simulink model "dianliuhuan"  (Simulink 8.5)
settings: Solver=ode23tb  StartTime=0.0  StopTime=5  RelTol=1e-3
libraries: powerlib x14, powerlib_extras x2
settings Model: Creator=Administrator  LastModifiedBy=佳君
settings DebuggingCC: SolverPrmCheckMsg=warning  FcnCallInpInsideContextMsg=UseLocalSettings  StrictBusMsg=Warning

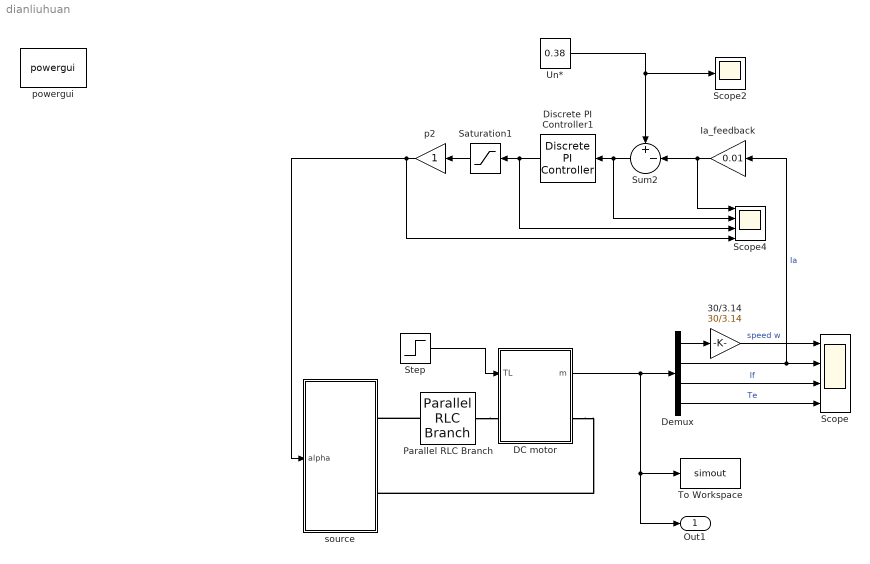
== system dianliuhuan ==
  30/3.14 : Gain  Gain=30/3.14
  DC motor : Subsystem
  Demux : Demux
  Discrete PI Controller1 : powerlib_extras/Discrete  Control Blocks/Discrete PI Controller  Kp=01  Ki=6  Par_Limits=[1e6 -1e6]  Init=0  Ts=50e-6
  Ia_feedback : Gain  Gain=0.01
  Parallel RLC Branch : powerlib/Elements/Parallel RLC Branch  LConnTagsString=a  RConnTagsString=__new0  BranchType=L  Resistance=1  Inductance=1e-3  SetiL0=off  InitialCurrent=0  Capacitance=1e-6  Setx0=off  InitialVoltage=0  Measurements=Branch voltage and current
  Saturation1 : Saturate  UpperLimit=10  LowerLimit=-10
  Scope : Scope  NumInputPorts=4
      settings: TimeRange=5  YMin=-0.1290027482477591~0~0.9166666666665609~0  YMax=2000~600~0.9166666666667626~1000
  Scope2 : Scope
      settings: YMin=0  YMax=13  SaveName=ScopeData2
  Scope4 : Scope  NumInputPorts=4
      settings: TimeRange=5  YMin=0~-5~-12~0  YMax=5.5~0.5~1~0.3  SaveName=ScopeData4
  Step : Step  Time=2  Before=50  After=100  SampleTime=0
  Sum2 : Sum  Inputs=+-|
  To Workspace : ToWorkspace  VariableName=simout  SaveFormat=Structure  SampleTime=-1
  Un* : Constant  Value=0.38
  p2 : Gain
  powergui : powerlib/powergui  Priority=1  SimulationMode=Continuous  SolverType=Tustin/Backward Euler (TBE)  SampleTime=50e-6  frequency=60  SPID=off  DisableSnubberDevices=off  DisableRonSwitches=off  DisableVfSwitches=off  SwTol=0  DisplayEquations=off  Interpol=off  methode=off  Ts=0  FunctionMessages=off  echomessages=off  HookPort=off  EnableUseOfTLC=off  x0status=blocks  frequencyindice=0  Pbase=100e6  ErrMax=1e-4  Iterations=50  UnitsV=kV  UnitsW=MW  buscounter=0  RestoreLinks=warning  ResistiveCurrentMeasurement=off  Frange=[0:2:500]  Ylog=off  Xlog=on  ShowGrid=off  save=off  variable=ZData  structure=0  ZoomFFT=on  StartTime=0.0  cycles=1  DisplayStyle=1  fundamental=60  FreqAxis=off  MaxFrequency=1000  frequencyindicesteady=1  RmsSteady=1  display=off
  source : Subsystem
  Out1 : Outport
  wires:
  DC motor/1(m) -> Demux/1, Out1/1, To Workspace/1
  Demux/2 -> Ia_feedback/1, Scope/2  "Ia"
  Demux/3 -> Scope/3  "If"
  Demux/4 -> Scope/4  "Te"
  Demux/1 -> 30/3.14/1
  30/3.14/1 -> Scope/1  "speed w"
  Step/1 -> DC motor/1(TL)
  Ia_feedback/1 -> Sum2/2, Scope4/1
  Sum2/1 -> Scope4/2, Discrete PI Controller1/1
  Saturation1/1 -> p2/1
  p2/1 -> Scope4/4, source/1(alpha)
  Un*/1 -> Sum2/1, Scope2/1
  Discrete PI Controller1/1 -> Scope4/3, Saturation1/1
  connections:
  Parallel RLC Branch/LConn1 -- source/RConn1
  Parallel RLC Branch/RConn1 -- DC motor/LConn1
  DC motor/RConn1 -- source/RConn2

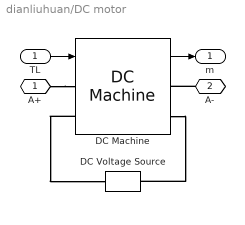
== system dianliuhuan/DC motor ==
  TL : Inport
  DC Machine : powerlib/Machines/DC Machine  PresetModel=No  MechanicalLoad=Torque TL  FieldType=Wound  ShowDetailedParameters=on  MeasurementBus=off  RLa=[0.6 0.012]  RLf=[240 120]  Laf=1.8  MachineConstant=Torque constant (N.m/A)  Ke=1.8  Kt=1.8  J=1  Bm=0  Tf=0  w0=0  Ifinit=0  TsPowergui=0  TsBlock=-1
  DC Voltage Source : powerlib/Electrical Sources/DC Voltage Source  Amplitude=220  Measurements=None
  A+ : PMIOPort  Port=1  Side=Left
  A- : PMIOPort  Port=2  Side=Right
  m : Outport
  wires:
  TL/1 -> DC Machine/1
  DC Machine/1 -> m/1
  connections:
  DC Machine/LConn2 -- DC Voltage Source/RConn1
  DC Machine/RConn2 -- DC Voltage Source/LConn1
  A+/RConn1 -- DC Machine/LConn1
  A-/RConn1 -- DC Machine/RConn1

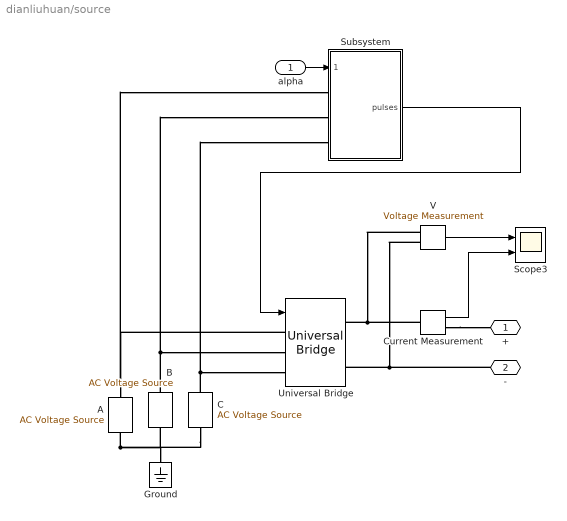
== system dianliuhuan/source ==
  alpha : Inport
  A : powerlib/Electrical Sources/AC Voltage Source  Amplitude=220  Phase=0  Frequency=50  SampleTime=0  Measurements=Voltage
  B : powerlib/Electrical Sources/AC Voltage Source  Amplitude=220  Phase=240  Frequency=50  SampleTime=0  Measurements=Voltage
  C : powerlib/Electrical Sources/AC Voltage Source  Amplitude=220  Phase=120  Frequency=50  SampleTime=0  Measurements=Voltage
  Current Measurement : powerlib/Measurements/Current Measurement  PhasorSimulation=off  OutputType=Complex  PSBequivalent=0
  Ground : powerlib/Elements/Ground  LConnTagsString=a
  Scope3 : Scope  NumInputPorts=2
      settings: YMin=-25~0  YMax=400~525
  Subsystem : Subsystem
  Universal Bridge : powerlib/Power Electronics/Universal Bridge  Arms=3  SnubberResistance=1e5  SnubberCapacitance=inf  Device=Thyristors  Ron=1e-3  Lon=0  ForwardVoltages="[  0  0  ]"  ForwardVoltage=0  GTOparameters=[ 10e-6 , 20e-6 ]  IGBTparameters=[ 1e-6 , 2e-6 ]  Measurements=None  Measurements_2=None  converterType=Rectifier
  V : powerlib/Measurements/Voltage Measurement  PhasorSimulation=off  OutputType=Complex  PSBequivalent=0
  + : PMIOPort  Port=1  Side=Right
  - : PMIOPort  Port=2  Side=Right
  wires:
  Subsystem/1(pulses) -> Universal Bridge/1
  alpha/1 -> Subsystem/1(alpha_deg)
  V/1 -> Scope3/1
  Current Measurement/1 -> Scope3/2
  connections:
  A/LConn1 -- C/LConn1 -- B/LConn1 -- Ground/LConn1
  A/RConn1 -- Subsystem/LConn1 -- Universal Bridge/LConn1
  B/RConn1 -- Subsystem/LConn2 -- Universal Bridge/LConn2
  C/RConn1 -- Subsystem/LConn3 -- Universal Bridge/LConn3
  V/LConn1 -- Current Measurement/LConn1 -- Universal Bridge/RConn1
  -/RConn1 -- Universal Bridge/RConn2 -- V/LConn2
  Current Measurement/RConn1 -- +/RConn1

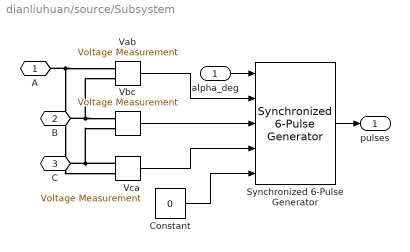
== system dianliuhuan/source/Subsystem ==
  alpha_deg : Inport
  Constant : Constant  Value=0
  Synchronized 6-Pulse Generator : powerlib_extras/Control  Blocks/Synchronized 6-Pulse Generator  freq=50  pwidth=10  Double_Pulse=off
  Vab : powerlib/Measurements/Voltage Measurement  PhasorSimulation=off  OutputType=Complex  PSBequivalent=0
  Vbc : powerlib/Measurements/Voltage Measurement  PhasorSimulation=off  OutputType=Complex  PSBequivalent=0
  Vca : powerlib/Measurements/Voltage Measurement  PhasorSimulation=off  OutputType=Complex  PSBequivalent=0
  A : PMIOPort  Port=1  Side=Left
  B : PMIOPort  Port=2  Side=Left
  C : PMIOPort  Port=3  Side=Left
  pulses : Outport
  wires:
  Vab/1 -> Synchronized 6-Pulse Generator/2
  Vbc/1 -> Synchronized 6-Pulse Generator/3
  Vca/1 -> Synchronized 6-Pulse Generator/4
  Constant/1 -> Synchronized 6-Pulse Generator/5
  alpha_deg/1 -> Synchronized 6-Pulse Generator/1
  Synchronized 6-Pulse Generator/1 -> pulses/1
  connections:
  A/RConn1 -- Vca/LConn2 -- Vab/LConn1
  B/RConn1 -- Vbc/LConn1 -- Vab/LConn2
  C/RConn1 -- Vca/LConn1 -- Vbc/LConn2
